simulink library "dspspect3"  (Simulink 8.2)
settings: Solver=ode45  SolverMode=SingleTasking  StartTime=0.0  StopTime=10.0  RelTol=1e-3
values from neighbouring files (symbols this model uses):
  D = D + B    [rebuffer_delay.m]
undefined symbols (not defined in the file or in its folder): dfilt, magnitude
libraries: dspmisc x6, dspspect3 x5, dspparest3 x4, dspxfrm3 x1, dsparch4 x1, dspsigattribs x1, dspsigops x1
settings Model: RequirementInfo=9  FPTRunName=Active  ForwardingTableString=||__slOldName__||dspspect3/Short-Time FFT||__slNewName__||dspspect3/Periodogram  Creator=don  LastModifiedBy=jibrahim  CovMetricSettings=d  ExtModeAutoUpdateStatusClock=off

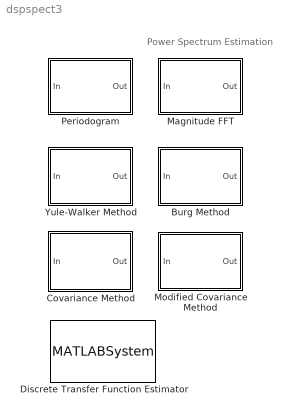
== system dspspect3 ==
  note: Power Spectrum Estimation
  Burg Method : Subsystem  mask(Burg Method){inheritOrd=off, ord=6, inheritFFT=off, fftsize=256, inheritTs=on, Ts=1}
      mask prompts: inheritOrd "Inherit estimation order from input dimensions"; ord "Estimation order:"; inheritFFT "Inherit FFT length from estimation order"; fftsize "FFT length:"; inheritTs "Inherit sample time from input"; Ts "Sample time of original time series:"
      mask help: Power spectral density estimation via Burg's method.
      mask init:
      | [xe,x,y]=dspblkburgmeth2('icon');
      | dspblkburgmeth2('init',inheritOrd,...
      |     inheritFFT,inheritTs,Ts);
      mask Help: eval('blocksethelp');
      mask Callback inheritOrd: dspblkburgmeth2('dynamic')
      mask Callback inheritFFT: dspblkburgmeth2('dynamic');
      mask Callback inheritTs: dspblkburgmeth2('dynamic');
      mask Display: text(-3,1.2,'Burg'); plot(-xe,0,xe,1.3,x,y)
  Covariance Method : Subsystem  mask(Covariance Method){ord=6, inheritFFT=off, fftsize=256, inheritTs=on, Ts=1}
      mask prompts: ord "Estimation order:"; inheritFFT "Inherit FFT length from estimation order"; fftsize "FFT length:"; inheritTs "Inherit sample time from input"; Ts "Sample time of original time series:"
      mask help: Power spectral density estimation via the covariance method.
      mask init:
      | [xe,x,y]=dspblkcovarmeth2('icon',ord,fftsize);
      | dspblkcovarmeth2('init',inheritFFT,inheritTs,Ts);
      mask Help: eval('blocksethelp');
      mask Callback inheritFFT: dspblkcovarmeth2('dynamic');
      mask Callback inheritTs: dspblkcovarmeth2('dynamic');
      mask Display: text(-3,1.2,'Cov AR'); plot(-xe,0,xe,1.3,x,y)
  Discrete Transfer Function Estimator : MATLABSystem  System=dsp.TransferFunctionEstimator  SpectralAverages=8  FFTLengthSource=Auto  FFTLength=128  Window=Hann  SidelobeAttenuation=60  FrequencyRange=twosided
      mask Type: dsp.TransferFunctionEstimator
      mask Display:
      | disp(['Discrete' char(10) 'Transfer Function' char(10) 'Estimator']);
      | port_label('input',1,'x');
      | port_label('input',2,'y');
      | port_label('output',1,'H');
  Magnitude FFT : Subsystem  mask(Magnitude FFT){mag_or_magsq=Magnitude squared, FFTImplementation=Auto, fftLenInherit=off, fftsize=256, WrapInput=on}
      mask prompts: mag_or_magsq "Output:"; FFTImplementation "FFT implementation:"; fftLenInherit "Inherit FFT length from input dimensions"; fftsize "FFT length:"; WrapInput "Wrap input data when FFT length is shorter than input length"
      mask help: Compute magnitude or magnitude-squared FFT of the input, with optional zero padding.
      mask init:
      | str=dspblkmagfft2('init');
      | dspblkmagfft2('update');
      mask Help: eval('blocksethelp');
      mask TypeOptions mag_or_magsq: Magnitude squared | Magnitude
      mask TypeOptions FFTImplementation: Auto | Radix-2 | FFTW
      mask Callback fftLenInherit: dspblkmagfft2;
      mask Display: disp(str,'texmode','on');
  Modified Covariance Method : Subsystem  mask(Modified Covariance Method){ord=6, inheritFFT=off, fftsize=256, inheritTs=on, Ts=1}
      mask prompts: ord "Estimation order:"; inheritFFT "Inherit FFT length from estimation order"; fftsize "FFT length:"; inheritTs "Inherit sample time from input"; Ts "Sample time of original time series:"
      mask help: Power spectral density estimation via the modified covariance method.
      mask init:
      | [xe,x,y]=dspblkmodcovmeth2('icon',ord, fftsize);
      | dspblkmodcovmeth2('init',inheritFFT,inheritTs,Ts);
      mask Help: eval('blocksethelp');
      mask Callback inheritFFT: dspblkmodcovmeth2('dynamic');
      mask Callback inheritTs: dspblkmodcovmeth2('dynamic');
      mask Display: text(-3,1.2,'MCov AR'); plot(-xe,0,xe,1.3,x,y)
  Periodogram : Subsystem  mask(Periodogram){measurement=Power spectral density, wintype=Hamming, Rs=50, beta=5, winsamp=Symmetric, FFTImplementation=Auto, inheritFFT=off, fftsize=256, navg=4, inheritTs=on, Ts=1}
      mask prompts: wintype "Window:"; Rs "Stopband attenuation in dB:"; winsamp "Window sampling:"; FFTImplementation "FFT implementation:"; inheritFFT "Inherit FFT length from input dimensions"; fftsize "FFT length:"; navg "Number of spectral averages:"; inheritTs "Inherit sample time from input"; Ts "Sample time of original time series:"
      mask help: Power spectral density and mean-square power spectrum estimation via the periodogram method and Welch's averaged, modified periodogram method.
      mask init:
      | [xe,x,y,iconStr]=dspblkshorttimefft2('icon',navg);
      | dspblkshorttimefft2('init',measurement,...
      |     inheritFFT,inheritTs,navg,Ts);
      mask Help: eval('blocksethelp');
      mask TypeOptions measurement: Power spectral density | Mean-square spectrum
      mask Callback measurement: dspblkshorttimefft2('dynamic');
      mask TypeOptions wintype: Bartlett | Blackman | Boxcar | Chebyshev | Hamming | Hann | Hanning | Kaiser | Triang
      mask Callback wintype: dspblkshorttimefft2('dynamic');
      mask TypeOptions winsamp: Symmetric | Periodic
      mask TypeOptions FFTImplementation: Auto | Radix-2 | FFTW
      mask Callback inheritFFT: dspblkshorttimefft2('dynamic');
      mask Callback inheritTs: dspblkshorttimefft2('dynamic');
      mask Display:
      | text(-3,1.15,iconStr);
      | plot((-xe),0,xe,1.3,x,y)
  Yule-Walker Method : Subsystem  mask(Yule-Walker Method){inheritOrd=off, ord=6, inheritFFT=off, fftsize=256, inheritTs=on, Ts=1}
      mask prompts: inheritOrd "Inherit estimation order from input dimensions"; ord "Estimation order:"; inheritFFT "Inherit FFT length from estimation order"; fftsize "FFT length:"; inheritTs "Inherit sample time from input"; Ts "Sample time of original time series:"
      mask help: Power spectral density estimation via Yule-Walker's method.
      mask init:
      | [xe,x,y]=dspblkyulewalkmeth2('icon');
      | dspblkyulewalkmeth2('init',inheritOrd,...
      |     inheritFFT,inheritTs, Ts);
      mask Help: eval('blocksethelp');
      mask Callback inheritOrd: dspblkyulewalkmeth2('dynamic');
      mask Callback inheritFFT: dspblkyulewalkmeth2('dynamic');
      mask Callback inheritTs: dspblkyulewalkmeth2('dynamic');
      mask Display: text(-3,1.2,'Yule AR'); plot(-xe,0,xe,1.3,x,y)

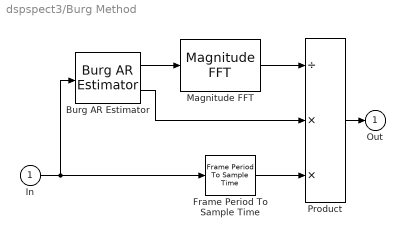
== system dspspect3/Burg Method ==
  In : Inport
  Burg AR Estimator : dspparest3/Burg AR Estimator  fcn=A  inheritOrder=off  ord=ord
  Frame Period To Sample Time : dspmisc/Frame Period To Sample Time
  Magnitude FFT : dspspect3/Magnitude FFT  mag_or_magsq=Magnitude squared  FFTImplementation=Auto  fftLenInherit=off  fftsize=fftsize  WrapInput=on
  Product : Product  Inputs=/**  SaturateOnIntegerOverflow=on  InputSameDT=on  OutDataTypeStr=Inherit: Same as first input
  Out : Outport  InitialOutput=0
  wires:
  In/1 -> Burg AR Estimator/1, Frame Period To Sample Time/1
  Burg AR Estimator/1 -> Magnitude FFT/1
  Magnitude FFT/1 -> Product/1
  Burg AR Estimator/2 -> Product/2
  Product/1 -> Out/1
  Frame Period To Sample Time/1 -> Product/3

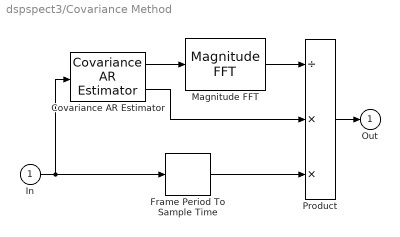
== system dspspect3/Covariance Method ==
  In : Inport
  Covariance AR Estimator : dspparest3/Covariance AR Estimator  P=ord
  Frame Period To Sample Time : dspmisc/Frame Period To Sample Time
  Magnitude FFT : dspspect3/Magnitude FFT  mag_or_magsq=Magnitude squared  FFTImplementation=Auto  fftLenInherit=off  fftsize=fftsize  WrapInput=on
  Product : Product  Inputs=/**  SaturateOnIntegerOverflow=on  InputSameDT=on  OutDataTypeStr=Inherit: Same as first input
  Out : Outport  InitialOutput=0
  wires:
  Magnitude FFT/1 -> Product/1
  Product/1 -> Out/1
  Covariance AR Estimator/1 -> Magnitude FFT/1
  Covariance AR Estimator/2 -> Product/2
  In/1 -> Covariance AR Estimator/1, Frame Period To Sample Time/1
  Frame Period To Sample Time/1 -> Product/3

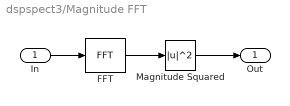
== system dspspect3/Magnitude FFT ==
  In : Inport
  FFT : dspxfrm3/FFT  CompMethod=Table lookup  TableOpt=NEW  TableOptActive=Speed  BitRevOrder=off  InheritFFTLength=off  FFTLength=fftsize  WrapInput=on  RowConvenienceOn=off  FFTImplementation=Auto  SkipNorm=off  firstCoeffDataTypeStr=Inherit: Same word length as input  firstCoeffLastDataTypeStr=Inherit: Same word length as input  outputMin=[]  outputMax=[]  roundingMode=Floor  overflowMode=off
  Magnitude Squared : Math  Operator=magnitude^2  SaturateOnIntegerOverflow=on  OutDataTypeStr=Inherit: Inherit via internal rule
  Out : Outport
  wires:
  Magnitude Squared/1 -> Out/1
  In/1 -> FFT/1
  FFT/1 -> Magnitude Squared/1

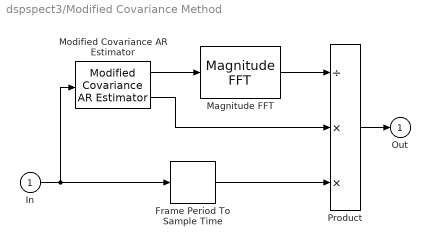
== system dspspect3/Modified Covariance Method ==
  In : Inport
  Frame Period To Sample Time : dspmisc/Frame Period To Sample Time
  Magnitude FFT : dspspect3/Magnitude FFT  mag_or_magsq=Magnitude squared  FFTImplementation=Auto  fftLenInherit=off  fftsize=fftsize  WrapInput=on
  Modified Covariance AR Estimator : dspparest3/Modified Covariance AR Estimator  P=ord
  Product : Product  Inputs=/**  SaturateOnIntegerOverflow=on  InputSameDT=on  OutDataTypeStr=Inherit: Same as first input
  Out : Outport  InitialOutput=0
  wires:
  In/1 -> Modified Covariance AR Estimator/1, Frame Period To Sample Time/1
  Modified Covariance AR Estimator/2 -> Product/2
  Modified Covariance AR Estimator/1 -> Magnitude FFT/1
  Product/1 -> Out/1
  Magnitude FFT/1 -> Product/1
  Frame Period To Sample Time/1 -> Product/3

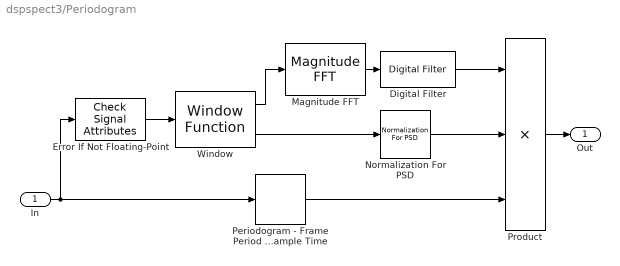
== system dspspect3/Periodogram ==
  In : Inport
  Digital Filter : dsparch4/Digital Filter  TypePopup=FIR (all zeros)  IIRFiltStruct=Direct form II transposed  AllPoleFiltStruct=Direct form  FIRFiltStruct=Direct form  CoeffSource=Specify via dialog  NumCoeffs=ones(navg,1)/navg  DenCoeffs=[1 0.1]  BiQuadCoeffs=[1 0.3 0.4 1 0.1 0.2]  LatticeCoeffs=[0.2 0.4]  denIgnore=on  FiltPerSampPopup=One filter per frame  IC=0  ICnum=0  ICden=0  roundingMode=Floor  overflowMode=off  ScaleValues=1  scaleValueFracLength=14  stageInFracLength=15  stageOutFracLength=15  FilterSource=Specify via dialog  dfiltObjectName=dfilt.dffir([1 2 1])
  Error If Not Floating-Point : dspsigattribs/Check Signal Attributes  SigAttribCheckMethod=Does not match attributes exactly  Complexity=Ignore  Frame=Ignore  DimsCheckMethod=Ignore  Dimensions=1-D  DatatypeCheckMethod=Is...  DatatypeGeneral=Floating-point  DtypeFloatSpecific=Any floating-point  DtypeFixedSpecific=Any fixed-point  DtypeIntSpecific=Any integer  SampleMode=Ignore
  Magnitude FFT : dspspect3/Magnitude FFT  mag_or_magsq=Magnitude squared  FFTImplementation=Auto  fftLenInherit=off  fftsize=fftsize  WrapInput=on
  Normalization For PSD : dspmisc/Normalization For PSD
  Periodogram - Frame Period To Sample Time : dspmisc/Periodogram - Frame Period To Sample Time
  Product : Product  Inputs=***  SaturateOnIntegerOverflow=on  InputSameDT=on  OutDataTypeStr=Inherit: Same as first input
  Window : dspsigops/Window Function  winmode=Generate and apply window  wintype=Hamming  sampmode=Continuous  samptime=1  N=64  Rs=Rs  beta=beta  winsamp=Symmetric  UserWindow=hamming  OptParams=off  UserParams={1.0}  RowConvenienceOn=off  dataType=double  isSigned=on  wordLen=16  udDataType=sfix(16)  fracBitsMode=Best precision  numFracBits=15  roundingMode=Floor  overflowMode=off  numSidelobes=4  sidelobeLevel=-30
      settings: additionalParams=on
  Out : Outport  InitialOutput=0
  wires:
  In/1 -> Error If Not Floating-Point/1, Periodogram - Frame Period To Sample Time/1
  Magnitude FFT/1 -> Digital Filter/1
  Window/1 -> Magnitude FFT/1
  Product/1 -> Out/1
  Digital Filter/1 -> Product/1
  Normalization For PSD/1 -> Product/2
  Window/2 -> Normalization For PSD/1
  Error If Not Floating-Point/1 -> Window/1
  Periodogram - Frame Period To Sample Time/1 -> Product/3

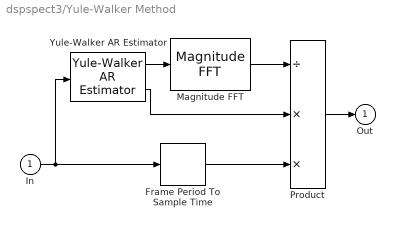
== system dspspect3/Yule-Walker Method ==
  In : Inport
  Frame Period To Sample Time : dspmisc/Frame Period To Sample Time
  Magnitude FFT : dspspect3/Magnitude FFT  mag_or_magsq=Magnitude squared  FFTImplementation=Auto  fftLenInherit=off  fftsize=fftsize  WrapInput=on
  Product : Product  Inputs=/**  SaturateOnIntegerOverflow=on  InputSameDT=on  OutDataTypeStr=Inherit: Same as first input
  Yule-Walker AR Estimator : dspparest3/Yule-Walker AR Estimator  ywArOutType=A  inheritOrder=off  ord=ord
  Out : Outport  InitialOutput=0
  wires:
  Product/1 -> Out/1
  Yule-Walker AR Estimator/1 -> Magnitude FFT/1
  Magnitude FFT/1 -> Product/1
  Yule-Walker AR Estimator/2 -> Product/2
  In/1 -> Yule-Walker AR Estimator/1, Frame Period To Sample Time/1
  Frame Period To Sample Time/1 -> Product/3
